simulink model "Prob1"  (R2020b)
settings: Solver=VariableStepAuto  StartTime=0.0  StopTime=10.0  RelTol=1e-3
model workspace (MAT data in the model file):
  b = Simulink.Parameter
  b.Value = 50
  b.DataType = 'auto'
  b.Dimensions = [1 1]
  k1 = Simulink.Parameter
  k1.Value = 50
  k1.DataType = 'auto'
  k1.Dimensions = [1 1]
  k12 = Simulink.Parameter
  k12.DataType = 'auto'
  k12.Dimensions = [0 0]
  m1 = Simulink.Parameter
  m1.Value = 100
  m1.DataType = 'auto'
  m1.Dimensions = [1 1]
  m2 = Simulink.Parameter
  m2.DataType = 'auto'
  m2.Dimensions = [0 0]
settings Model: Creator=shoun  LastModifiedBy=shoun

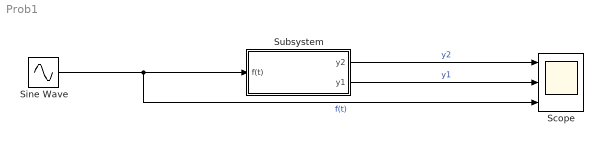
== system Prob1 ==
  Scope : Scope  NumInputPorts=3
  Sine Wave : Sin  SampleTime=0
  Subsystem : Subsystem  mask{m2=0, k12=0}
  wires:
  Sine Wave/1 -> Scope/3, Subsystem/1(f(t))  "f(t)"
  Subsystem/1(y2) -> Scope/1  "y2"
  Subsystem/2(y1) -> Scope/2  "y1"

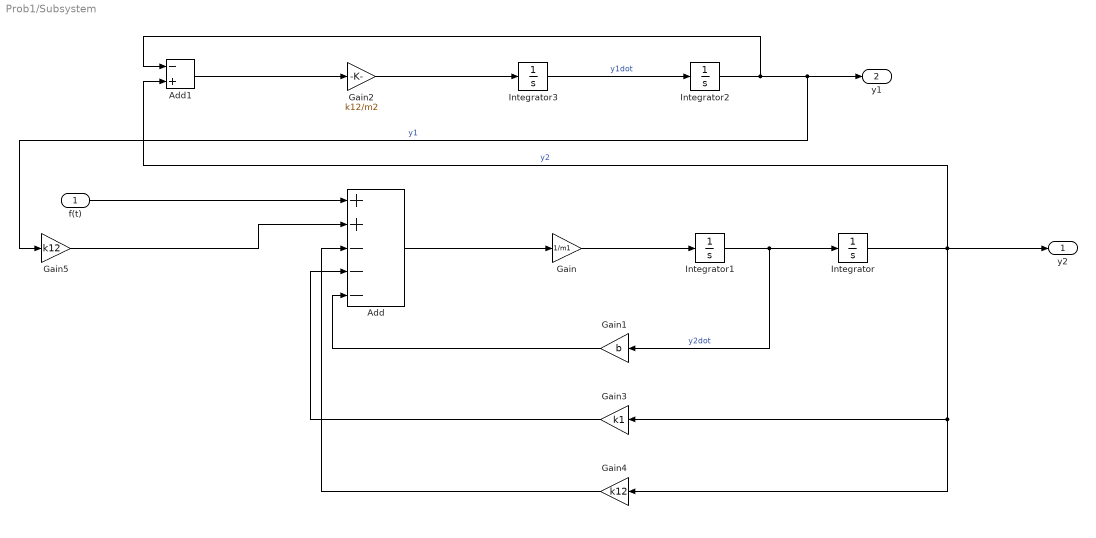
== system Prob1/Subsystem ==
  f(t) : Inport
  Add : Sum  Inputs=++---
  Add1 : Sum  Inputs=-+
  Gain : Gain  Gain=1/m1
  Gain1 : Gain  Gain=b
  Gain2 : Gain  Gain=k12/m2
  Gain3 : Gain  Gain=k1
  Gain4 : Gain  Gain=k12
  Gain5 : Gain  Gain=k12
  Integrator{,1..3} (4 alike) : Integrator
  y2 : Outport
  y1 : Outport  Port=2
  wires:
  f(t)/1 -> Add/1
  Gain5/1 -> Add/2
  Add/1 -> Gain/1
  Gain/1 -> Integrator1/1
  Integrator1/1 -> Gain1/1, Integrator/1  "y2dot"
  Add1/1 -> Gain2/1
  Gain2/1 -> Integrator3/1
  Integrator3/1 -> Integrator2/1  "y1dot"
  Integrator2/1 -> Add1/1, Gain5/1, y1/1  "y1"
  Gain1/1 -> Add/5
  Gain3/1 -> Add/4
  Gain4/1 -> Add/3
  Integrator/1 -> Gain3/1, Gain4/1, Add1/2, y2/1  "y2"
